simulink model "Capstone_Sim"  (R2023b)
settings: Solver=VariableStepAuto  StartTime=0.0  StopTime=10.0  RelTol=1e-3
values from neighbouring files (symbols this model uses):
  A_membrane = 0.01    [Capstone_Model.m]    (also in Capstone_Model_V2.m)
  C_membrane = 100    [Capstone_Model.m]    (also in Capstone_Model_V2.m)
  d_on = .4    (= 0.4)    [Capstone_Model.m]
  Knegative = 1000    [Capstone_Model.m]
  Kpositive = 1000    [Capstone_Model.m]
  P_neg = -10000    [Capstone_Model.m]
  P_pos = 20000    [Capstone_Model.m]
  Q_in = 0.001    [Capstone_Model.m]
  Q_out = 0.00066    [Capstone_Model.m]
  V0 = 0.01    [Capstone_Model.m]    (also in Capstone_Model_V2.m = 0.0005)
settings Model: Creator=johny  LastModifiedBy=johny

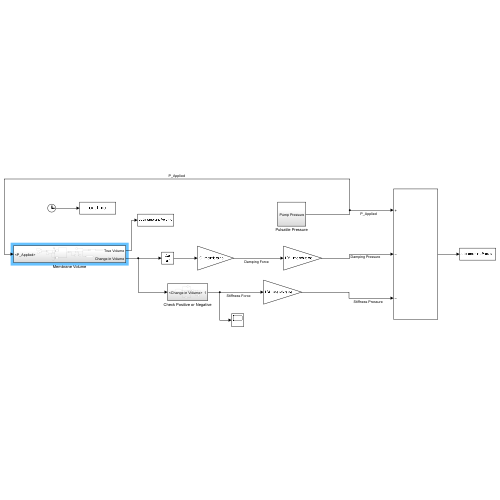
[thumbnail: Simulink's stored preview of the top-level diagram]
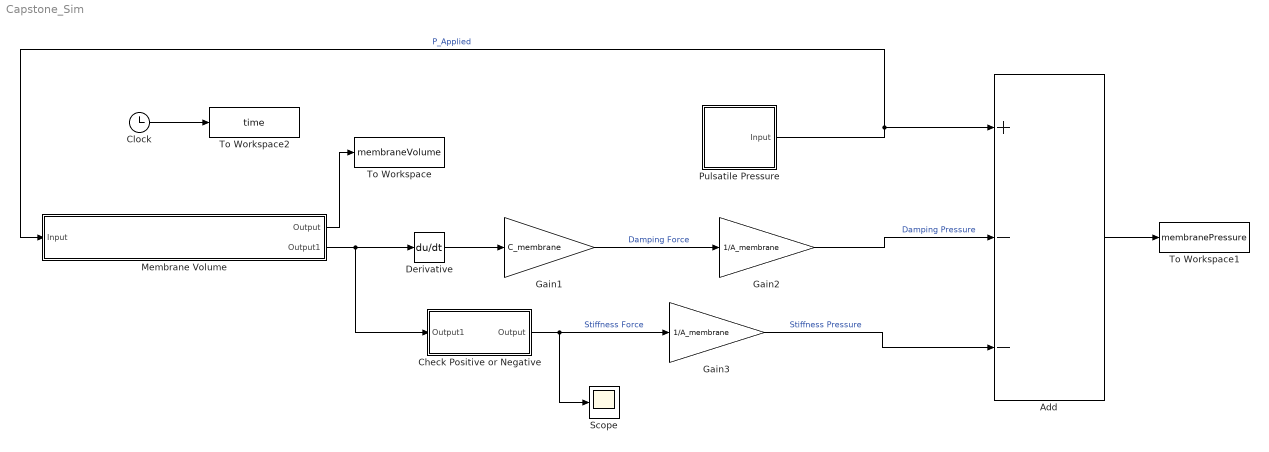
== system Capstone_Sim ==
  Add : Sum  Inputs=+--
  Check Positive or Negative : Subsystem
  Clock : Clock
  Derivative : Derivative
  Gain1 : Gain  Gain=C_membrane
  Gain2 : Gain  Gain=1/A_membrane
  Gain3 : Gain  Gain=1/A_membrane
  Membrane Volume : Subsystem
  Pulsatile Pressure : Subsystem
  Scope : Scope
  To Workspace : ToWorkspace  VariableName=membraneVolume  SampleTime=-1
  To Workspace1 : ToWorkspace  VariableName=membranePressure  SampleTime=-1
  To Workspace2 : ToWorkspace  VariableName=time  SampleTime=-1
  wires:
  Membrane Volume/2(Output1) -> Check Positive or Negative/1(Output1), Derivative/1
  Derivative/1 -> Gain1/1
  Gain1/1 -> Gain2/1  "Damping Force"
  Pulsatile Pressure/1(Input) -> Add/1, Membrane Volume/1(Input)  "P_Applied"
  Gain2/1 -> Add/2  "Damping Pressure"
  Gain3/1 -> Add/3  "Stiffness Pressure"
  Membrane Volume/1(Output) -> To Workspace/1
  Add/1 -> To Workspace1/1
  Clock/1 -> To Workspace2/1
  Check Positive or Negative/1(Output) -> Scope/1, Gain3/1  "Stiffness Force"

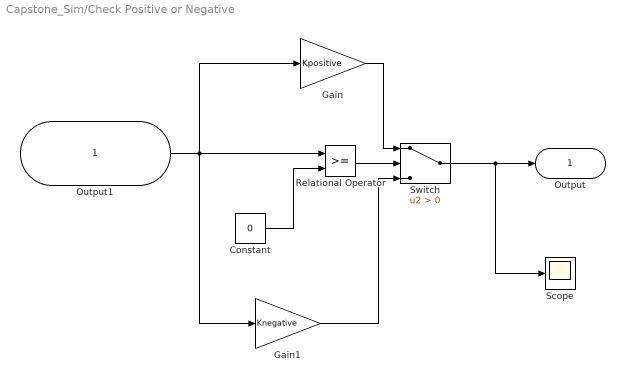
== system Capstone_Sim/Check Positive or Negative ==
  Output1 : Inport
  Constant : Constant  Value=0
  Gain : Gain  Gain=Kpositive
  Gain1 : Gain  Gain=Knegative
  Relational Operator : RelationalOperator  OutDataTypeStr=boolean  RndMeth=Simplest  InputSameDT=off
  Scope : Scope
  Switch : Switch  Criteria=u2 > Threshold  SaturateOnIntegerOverflow=off  InputSameDT=off
  Output : Outport
  wires:
  Output1/1 -> Gain/1, Gain1/1, Relational Operator/1
  Constant/1 -> Relational Operator/2
  Relational Operator/1 -> Switch/2
  Gain/1 -> Switch/1
  Gain1/1 -> Switch/3
  Switch/1 -> Scope/1, Output/1

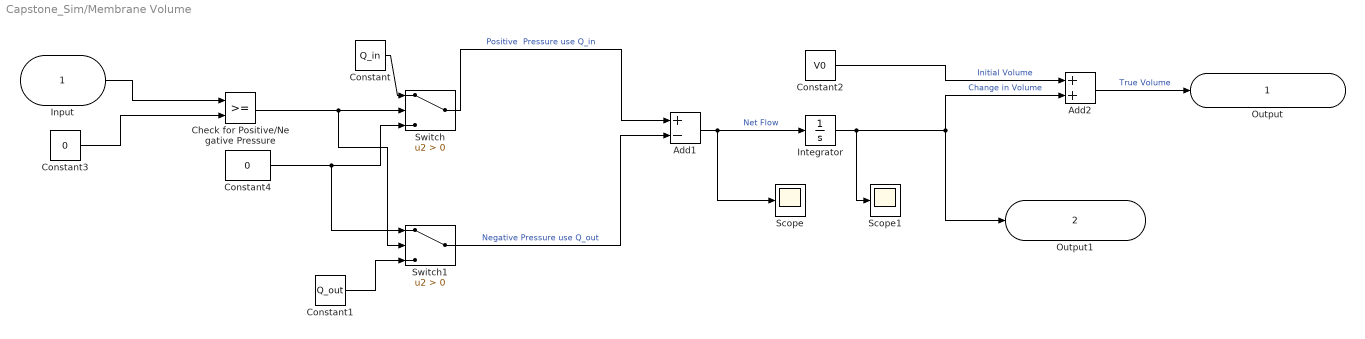
== system Capstone_Sim/Membrane Volume ==
  Input : Inport
  Add1 : Sum  Inputs=+-
  Add2 : Sum
  Check for Positive/Negative Pressure : RelationalOperator  OutDataTypeStr=boolean  RndMeth=Simplest  InputSameDT=off
  Constant : Constant  Value=Q_in
  Constant1 : Constant  Value=Q_out
  Constant2 : Constant  Value=V0
  Constant3 : Constant  Value=0
  Constant4 : Constant  Value=0
  Integrator : Integrator
  Scope : Scope
  Scope1 : Scope
  Switch : Switch  Criteria=u2 > Threshold  SaturateOnIntegerOverflow=off  InputSameDT=off
  Switch1 : Switch  Criteria=u2 > Threshold  SaturateOnIntegerOverflow=off  InputSameDT=off
  Output : Outport
  Output1 : Outport  Port=2
  wires:
  Add1/1 -> Scope/1, Integrator/1  "Net Flow"
  Constant2/1 -> Add2/1  "Initial Volume"
  Integrator/1 -> Scope1/1, Output1/1, Add2/2  "Change in Volume"
  Add2/1 -> Output/1  "True Volume"
  Input/1 -> Check for Positive/Negative Pressure/1
  Constant3/1 -> Check for Positive/Negative Pressure/2
  Check for Positive/Negative Pressure/1 -> Switch/2, Switch1/2
  Switch/1 -> Add1/1  "Positive  Pressure use Q_in"
  Constant/1 -> Switch/1
  Constant4/1 -> Switch/3, Switch1/1
  Constant1/1 -> Switch1/3
  Switch1/1 -> Add1/2  "Negative Pressure use Q_out"

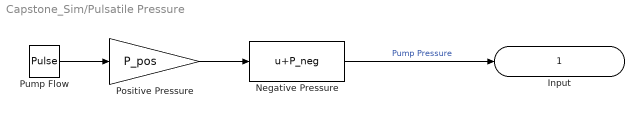
== system Capstone_Sim/Pulsatile Pressure ==
  Negative Pressure : Bias  Bias=P_neg  SaturateOnIntegerOverflow=off
  Positive Pressure : Gain  Gain=P_pos
  Pump Flow : DiscretePulseGenerator  PulseType=Time based  Period=.75  PulseWidth=d_on*100
  Input : Outport
  wires:
  Positive Pressure/1 -> Negative Pressure/1
  Pump Flow/1 -> Positive Pressure/1
  Negative Pressure/1 -> Input/1  "Pump Pressure"
